simulink model "SatelliteSimulink"  (R2020a)
settings: Solver=VariableStepAuto  StartTime=0.0  StopTime=10  RelTol=1e-3
libraries: cstblocks x1
settings Model: Creator=Strel  LastModifiedBy=Strel

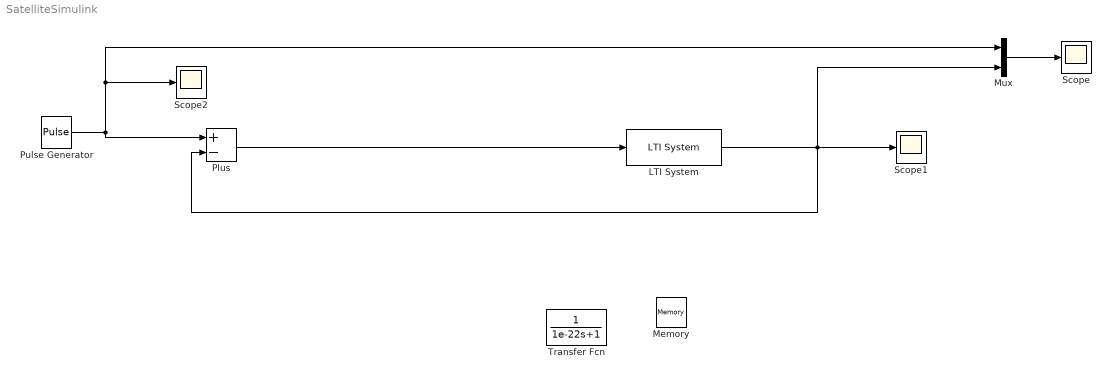
== system SatelliteSimulink ==
  LTI System : cstblocks/LTI System  sys=P_star_K  IC=[]
  Memory : Memory
  Mux : Mux  Inputs=2
  Plus : Sum  Inputs=+-
  Pulse Generator : DiscretePulseGenerator  PulseType=Time based  Amplitude=.1  Period=.2  PulseWidth=50
  Scope : Scope
  Scope1 : Scope
  Scope2 : Scope
  Transfer Fcn : TransferFcn  Denominator=[1e-22 1]
  wires:
  Plus/1 -> LTI System/1
  Mux/1 -> Scope/1
  Pulse Generator/1 -> Plus/1, Scope2/1, Mux/1
  LTI System/1 -> Plus/2, Scope1/1, Mux/2
